simulink model "mlinear"  (R2017a)
settings: Solver=VariableStepAuto  StartTime=0.0  StopTime=10.0  RelTol=1e-3
undefined symbols (not defined in the file or in its folder): veh
settings Model: Creator=yongyu  LastModifiedBy=yongyu

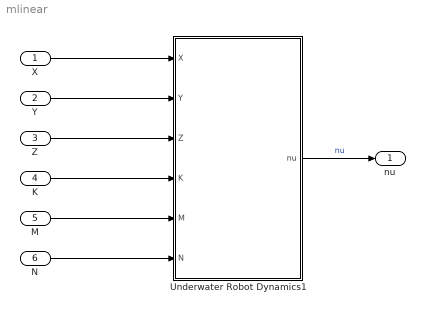
== system mlinear ==
  X : Inport
  Y : Inport  Port=2
  Z : Inport  Port=3
  K : Inport  Port=4
  M : Inport  Port=5
  N : Inport  Port=6
  Underwater Robot Dynamics1 : Subsystem
  nu : Outport
  wires:
  X/1 -> Underwater Robot Dynamics1/1(X)
  Underwater Robot Dynamics1/1(nu) -> nu/1  "nu"
  Y/1 -> Underwater Robot Dynamics1/2(Y)
  Z/1 -> Underwater Robot Dynamics1/3(Z)
  K/1 -> Underwater Robot Dynamics1/4(K)
  M/1 -> Underwater Robot Dynamics1/5(M)
  N/1 -> Underwater Robot Dynamics1/6(N)

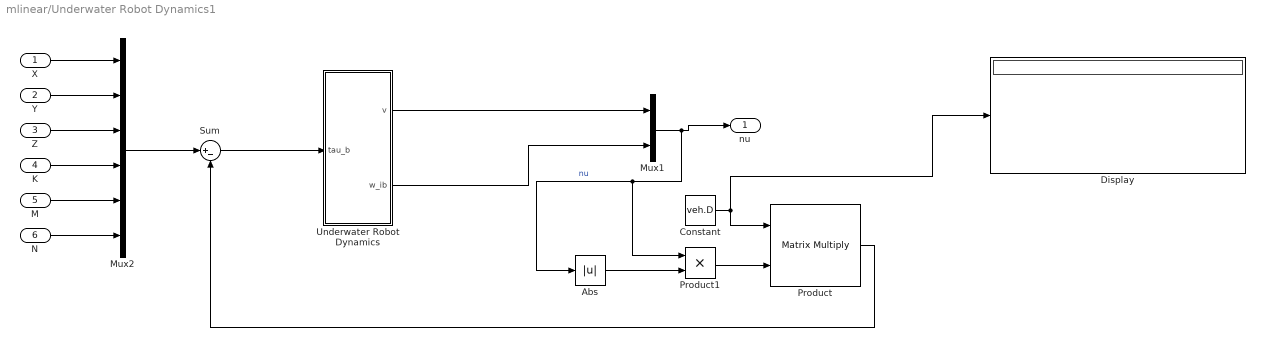
== system mlinear/Underwater Robot Dynamics1 ==
  X : Inport
  Y : Inport  Port=2
  Z : Inport  Port=3
  K : Inport  Port=4
  M : Inport  Port=5
  N : Inport  Port=6
  Abs : Abs
  Constant : Constant  Value=veh.D
  Display : Display
  Mux1 : Mux  Inputs=2
  Mux2 : Mux  Inputs=6
  Product : Product  Multiplication=Matrix(*)
  Product1 : Product
  Sum : Sum  Inputs=|+-
  "Underwater Robot Dynamics " : Subsystem
  nu : Outport
  wires:
  Mux1/1 -> Product1/1, Abs/1, nu/1  "nu"
  "Underwater Robot Dynamics "/2(w_ib) -> Mux1/2
  N/1 -> Mux2/6
  M/1 -> Mux2/5
  K/1 -> Mux2/4
  Z/1 -> Mux2/3
  Y/1 -> Mux2/2
  X/1 -> Mux2/1
  "Underwater Robot Dynamics "/1(v) -> Mux1/1
  Constant/1 -> Product/1, Display/1
  Mux2/1 -> Sum/1
  Sum/1 -> "Underwater Robot Dynamics "/1(tau_b)
  Product/1 -> Sum/2
  Abs/1 -> Product1/2
  Product1/1 -> Product/2

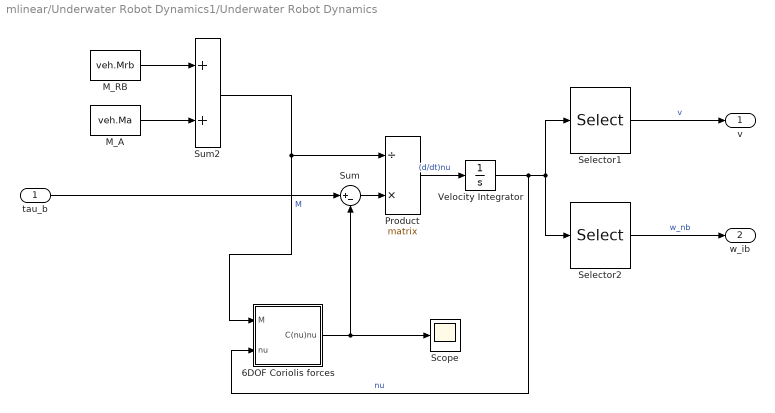
== system mlinear/Underwater Robot Dynamics1/Underwater Robot Dynamics  ==
  tau_b : Inport
  6DOF Coriolis forces : Subsystem
  M_A : Constant  Value=veh.Ma
  M_RB : Constant  Value=veh.Mrb
  Product : Product  Inputs=/*  Multiplication=Matrix(*)  SaturateOnIntegerOverflow=on  OutDataTypeStr=Inherit: Same as first input
  Scope : Scope
  Selector1 : Selector  InputPortWidth=6  IndexOptions=Index vector (dialog)  Indices=[1 2 3]  OutputSizes=1
  Selector2 : Selector  InputPortWidth=6  IndexOptions=Index vector (dialog)  Indices=[4 5 6]  OutputSizes=1
  Sum : Sum  Inputs=|+-
  Sum2 : Sum  SaturateOnIntegerOverflow=on
  Velocity Integrator : Integrator
  v : Outport
  w_ib : Outport  Port=2
  wires:
  M_RB/1 -> Sum2/1
  M_A/1 -> Sum2/2
  Sum2/1 -> Product/1, 6DOF Coriolis forces/1(M)  "M"
  Selector2/1 -> w_ib/1  "w_nb"
  Product/1 -> Velocity Integrator/1  "(d/dt)nu"
  6DOF Coriolis forces/1(C(nu)nu) -> Sum/2, Scope/1
  Sum/1 -> Product/2
  Selector1/1 -> v/1  "v"
  Velocity Integrator/1 -> 6DOF Coriolis forces/2(nu), Selector2/1, Selector1/1  "nu"
  tau_b/1 -> Sum/1

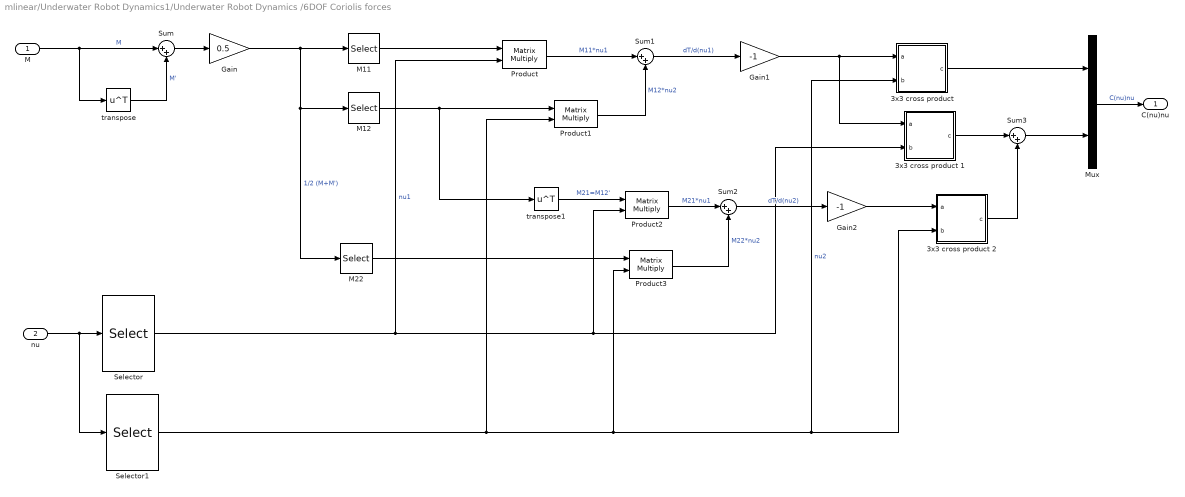
== system mlinear/Underwater Robot Dynamics1/Underwater Robot Dynamics /6DOF Coriolis forces ==
  M : Inport
  nu : Inport  Port=2
  3x3 cross product : Subsystem
  3x3 cross product 1 : Subsystem
  3x3 cross product 2 : Subsystem
  Gain : Gain  Gain=0.5  SaturateOnIntegerOverflow=on  OutDataTypeStr=Inherit: Same as input  ParamDataTypeStr=Inherit: Same as input
  Gain1 : Gain  Gain=-1  SaturateOnIntegerOverflow=on  OutDataTypeStr=Inherit: Same as input  ParamDataTypeStr=Inherit: Same as input
  Gain2 : Gain  Gain=-1  SaturateOnIntegerOverflow=on  OutDataTypeStr=Inherit: Same as input  ParamDataTypeStr=Inherit: Same as input
  M11 : Selector  NumberOfDimensions=2  InputPortWidth=3  IndexOptions=Index vector (dialog),Index vector (dialog)  Indices=[1 2 3],[1 2 3]  OutputSizes=1
  M12 : Selector  NumberOfDimensions=2  InputPortWidth=3  IndexOptions=Index vector (dialog),Index vector (dialog)  Indices=[1 2 3],[4 5 6]  OutputSizes=1
  M22 : Selector  NumberOfDimensions=2  InputPortWidth=3  IndexOptions=Index vector (dialog),Index vector (dialog)  Indices=[4 5 6],[4 5 6]  OutputSizes=1
  Mux : Mux  Inputs=2
  Product{,1..3} (4 alike) : Product  Multiplication=Matrix(*)  SaturateOnIntegerOverflow=on  OutDataTypeStr=Inherit: Same as first input
  Selector : Selector  InputPortWidth=6  IndexOptions=Index vector (dialog)  Indices=[1 2 3]  OutputSizes=1
  Selector1 : Selector  InputPortWidth=6  IndexOptions=Index vector (dialog)  Indices=[4 5 6]  OutputSizes=1
  Sum{,1..3} (4 alike) : Sum  Inputs=|++  SaturateOnIntegerOverflow=on
  transpose : Math  Operator=transpose  SaturateOnIntegerOverflow=on
  transpose1 : Math  Operator=transpose  SaturateOnIntegerOverflow=on
  C(nu)nu : Outport
  wires:
  transpose/1 -> Sum/2  "M'"
  Sum/1 -> Gain/1
  Gain/1 -> M22/1, M12/1, M11/1  "1/2 (M+M')"
  Selector/1 -> Product2/2, 3x3 cross product 1/2(b), Product/2  "nu1"
  Selector1/1 -> 3x3 cross product/2(b), 3x3 cross product 2/2(b), Product3/2, Product1/2  "nu2"
  M11/1 -> Product/1
  Product/1 -> Sum1/1  "M11*nu1"
  M12/1 -> transpose1/1, Product1/1
  Product1/1 -> Sum1/2  "M12*nu2"
  Sum1/1 -> Gain1/1  "dT/d(nu1)"
  transpose1/1 -> Product2/1  "M21=M12'"
  Product2/1 -> Sum2/1  "M21*nu1"
  M22/1 -> Product3/1
  Product3/1 -> Sum2/2  "M22*nu2"
  Sum2/1 -> Gain2/1  "dT/d(nu2)"
  Gain1/1 -> 3x3 cross product/1(a), 3x3 cross product 1/1(a)
  3x3 cross product/1(c) -> Mux/1
  Gain2/1 -> 3x3 cross product 2/1(a)
  3x3 cross product 1/1(c) -> Sum3/1
  3x3 cross product 2/1(c) -> Sum3/2
  Sum3/1 -> Mux/2
  Mux/1 -> C(nu)nu/1  "C(nu)nu"
  nu/1 -> Selector/1, Selector1/1
  M/1 -> transpose/1, Sum/1  "M"

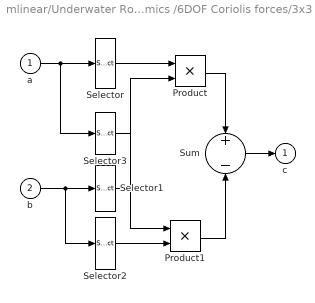
== system mlinear/Underwater Robot Dynamics1/Underwater Robot Dynamics /6DOF Coriolis forces/3x3 cross product ==
  a : Inport
  b : Inport  Port=2
  Product : Product  SaturateOnIntegerOverflow=on  InputSameDT=on  OutDataTypeStr=Inherit: Same as first input
  Product1 : Product  SaturateOnIntegerOverflow=on  InputSameDT=on  OutDataTypeStr=Inherit: Same as first input
  Selector : Selector  InputPortWidth=3  IndexOptions=Index vector (dialog)  Indices=[2 3 1]  OutputSizes=1
  Selector1 : Selector  InputPortWidth=3  IndexOptions=Index vector (dialog)  Indices=[3 1 2]  OutputSizes=1
  Selector2 : Selector  InputPortWidth=3  IndexOptions=Index vector (dialog)  Indices=[2 3 1]  OutputSizes=1
  Selector3 : Selector  InputPortWidth=3  IndexOptions=Index vector (dialog)  Indices=[3 1 2]  OutputSizes=1
  Sum : Sum  Inputs=+|-  SaturateOnIntegerOverflow=on  InputSameDT=on  OutDataTypeStr=Inherit: Same as first input
  c : Outport  InitialOutput=0
  wires:
  Selector3/1 -> Product1/1
  Selector2/1 -> Product1/2
  Product1/1 -> Sum/2
  Selector1/1 -> Product/2
  Product/1 -> Sum/1
  a/1 -> Selector3/1, Selector/1
  Selector/1 -> Product/1
  b/1 -> Selector2/1, Selector1/1
  Sum/1 -> c/1

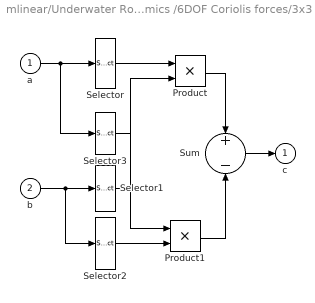
== system mlinear/Underwater Robot Dynamics1/Underwater Robot Dynamics /6DOF Coriolis forces/3x3 cross product 1 ==
  a : Inport
  b : Inport  Port=2
  Product : Product  SaturateOnIntegerOverflow=on  InputSameDT=on  OutDataTypeStr=Inherit: Same as first input
  Product1 : Product  SaturateOnIntegerOverflow=on  InputSameDT=on  OutDataTypeStr=Inherit: Same as first input
  Selector : Selector  InputPortWidth=3  IndexOptions=Index vector (dialog)  Indices=[2 3 1]  OutputSizes=1
  Selector1 : Selector  InputPortWidth=3  IndexOptions=Index vector (dialog)  Indices=[3 1 2]  OutputSizes=1
  Selector2 : Selector  InputPortWidth=3  IndexOptions=Index vector (dialog)  Indices=[2 3 1]  OutputSizes=1
  Selector3 : Selector  InputPortWidth=3  IndexOptions=Index vector (dialog)  Indices=[3 1 2]  OutputSizes=1
  Sum : Sum  Inputs=+|-  SaturateOnIntegerOverflow=on  InputSameDT=on  OutDataTypeStr=Inherit: Same as first input
  c : Outport  InitialOutput=0
  wires:
  Selector3/1 -> Product1/1
  Selector2/1 -> Product1/2
  Product1/1 -> Sum/2
  Selector1/1 -> Product/2
  Product/1 -> Sum/1
  a/1 -> Selector3/1, Selector/1
  Selector/1 -> Product/1
  b/1 -> Selector2/1, Selector1/1
  Sum/1 -> c/1

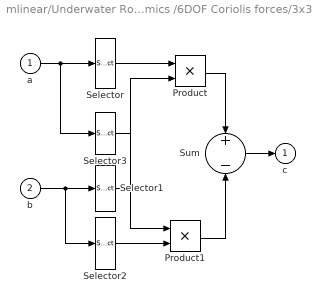
== system mlinear/Underwater Robot Dynamics1/Underwater Robot Dynamics /6DOF Coriolis forces/3x3 cross product 2 ==
  a : Inport
  b : Inport  Port=2
  Product : Product  SaturateOnIntegerOverflow=on  InputSameDT=on  OutDataTypeStr=Inherit: Same as first input
  Product1 : Product  SaturateOnIntegerOverflow=on  InputSameDT=on  OutDataTypeStr=Inherit: Same as first input
  Selector : Selector  InputPortWidth=3  IndexOptions=Index vector (dialog)  Indices=[2 3 1]  OutputSizes=1
  Selector1 : Selector  InputPortWidth=3  IndexOptions=Index vector (dialog)  Indices=[3 1 2]  OutputSizes=1
  Selector2 : Selector  InputPortWidth=3  IndexOptions=Index vector (dialog)  Indices=[2 3 1]  OutputSizes=1
  Selector3 : Selector  InputPortWidth=3  IndexOptions=Index vector (dialog)  Indices=[3 1 2]  OutputSizes=1
  Sum : Sum  Inputs=+|-  SaturateOnIntegerOverflow=on  InputSameDT=on  OutDataTypeStr=Inherit: Same as first input
  c : Outport  InitialOutput=0
  wires:
  Selector3/1 -> Product1/1
  Selector2/1 -> Product1/2
  Product1/1 -> Sum/2
  Selector1/1 -> Product/2
  Product/1 -> Sum/1
  a/1 -> Selector3/1, Selector/1
  Selector/1 -> Product/1
  b/1 -> Selector2/1, Selector1/1
  Sum/1 -> c/1
